simulink subsystem "Charger"  (R2024b)
settings: Solver=VariableStepAuto  StartTime=0.0  StopTime=10.0  RelTol=1e-3
undefined symbols (not defined in the file or in its folder): battery
libraries: fl_lib x2, BatteryCurrentManagement x1, nesl_utility x1
Description:
  | Charger (No Thermal)
  | 
  | ⚡ Main Features:
  | - Constant-current, constant-voltage (CC–CV) charging control
  | - Inputs: relay command, battery cell voltage, and charging state
  | - Generates charging current and applies to HV bus
  | - Simplified model without thermal dynamics
  | - Focused on electrical charging behavior
  | 
  | 📤 Outputs: Charging Current, HV Power
  | 
  | 📌 Use Case: Fast simulations of charging process without thermal coupling
settings Model: Creator=jjha  LastModifiedBy=jjha

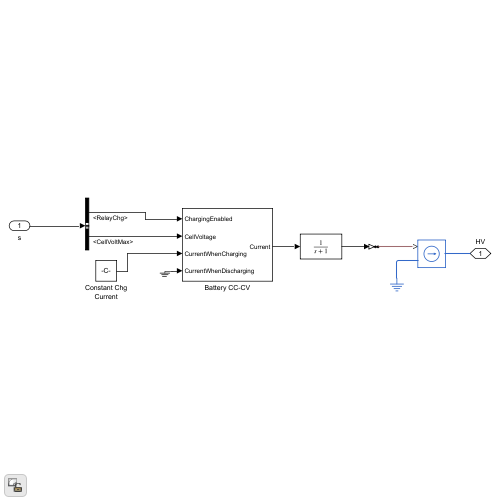
[thumbnail: Simulink's stored preview of the top-level diagram]
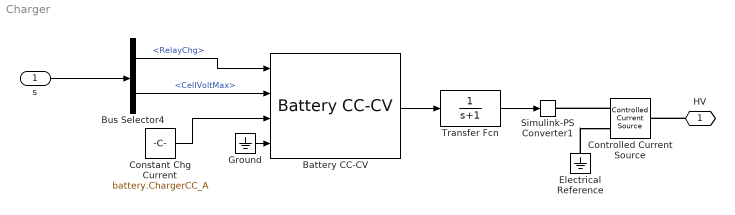
== system Charger ==
  s : Inport
  Battery CC-CV : BatteryCurrentManagement/Battery CC-CV  MaxCellVoltage=battery.ChargeMaxVolt  Kp=battery.ChargeKp  Ki=battery.ChargerKi  Kaw=battery.ChargerKaw  Kt=1  Ts=-1
  Bus Selector4 : BusSelector  OutputSignals=Batt.Relay.RelayChg,Batt.BattSensor.CellVoltMax
  Constant Chg Current : Constant  Value=battery.ChargerCC_A
  Controlled Current Source : fl_lib/Electrical/Electrical Sources/Controlled Current Source
  Electrical Reference : fl_lib/Electrical/Electrical Elements/Electrical Reference
  Ground : Ground
  Simulink-PS Converter1 : nesl_utility/Simulink-PS Converter  PhysicalDomain=network_engine_domain  SubClassName=ps_input  LeftPortType=input  RightPortType=output  PseudoPeriodic=off  Frequencies=[]  NoiseDistribution=none  NoiseParameters=[]  Unit=A  AffineConversion=off  FilteringAndDerivatives=filter  SimscapeFilterOrder=2  InputFilterTimeConstant=0.01  UdotUserProvided=0
  Transfer Fcn : TransferFcn  Denominator=[1 1]
  HV : PMIOPort  Side=Left
  wires:
  Transfer Fcn/1 -> Simulink-PS Converter1/1
  Constant Chg Current/1 -> Battery CC-CV/3
  Bus Selector4/2 -> Battery CC-CV/2  "<CellVoltMax>"
  Bus Selector4/1 -> Battery CC-CV/1  "<RelayChg>"
  Battery CC-CV/1 -> Transfer Fcn/1
  Ground/1 -> Battery CC-CV/4
  s/1 -> Bus Selector4/1
  connections:
  Electrical Reference/LConn1 -- Controlled Current Source/RConn2
  HV/RConn1 -- Controlled Current Source/LConn1
  Controlled Current Source/RConn1 -- Simulink-PS Converter1/RConn1
